simulink model "ideal_defence_zda"  (R2022a)
settings: Solver=VariableStepAuto  StartTime=0.0  StopTime=6  RelTol=1e-3
values from neighbouring files (symbols this model uses):
  A = [zeros(3, 3) eye(3) ... (first row only)    [ideal_defence_zda.m]
  B = [zeros(3, 3); inv(M)]    [ideal_defence_zda.m]
  b = Cp*(A^(r-1))*Bp    [ideal_defence_zda.m]
  H0 = Cp*(A^r)*T0_inv    [ideal_defence_zda.m]
  K = Cp*(A^r)*T1_inv    [ideal_defence_zda.m]
  K0 = [-9 -6]    [ideal_defence_zda.m]
  Ka = (-1)*acker(F0, G0a, [1/tau1 1/tau1 1/tau1 1/tau1])    [ideal_defence_zda.m]
  omega20 = 1.3e-2    (= 0.013)    [ideal_defence_zda.m]
  T0 = [1 0 0 0 0 0 ... (first row only)    [ideal_defence_zda.m]
  T1 = [Cp; Cp*A]    [ideal_defence_zda.m]
settings Model: Creator=edebi  LastModifiedBy=edebi

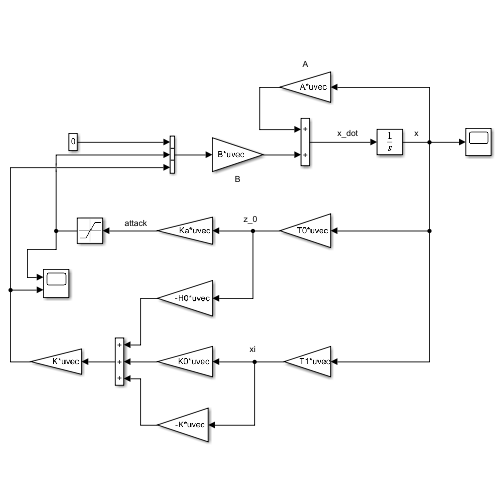
[thumbnail: Simulink's stored preview of the top-level diagram]
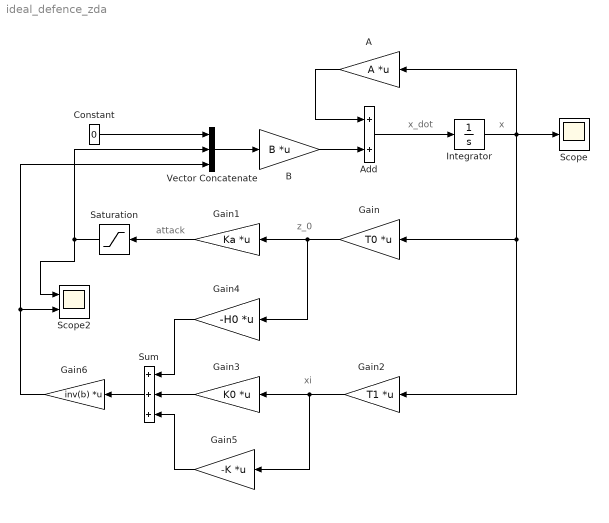
== system ideal_defence_zda ==
  note: xi
  note: attack
  note: z_0
  note: x
  note: x_dot
  A : Gain  Gain=A  Multiplication=Matrix(K*u) (u vector)
  Add : Sum
  B : Gain  Gain=B  Multiplication=Matrix(K*u) (u vector)
  Constant : Constant  Value=0
  Gain : Gain  Gain=T0  Multiplication=Matrix(K*u) (u vector)
  Gain1 : Gain  Gain=Ka  Multiplication=Matrix(K*u) (u vector)
  Gain2 : Gain  Gain=T1  Multiplication=Matrix(K*u) (u vector)
  Gain3 : Gain  Gain=K0  Multiplication=Matrix(K*u) (u vector)
  Gain4 : Gain  Gain=-H0  Multiplication=Matrix(K*u) (u vector)
  Gain5 : Gain  Gain=-K  Multiplication=Matrix(K*u) (u vector)
  Gain6 : Gain  Gain=inv(b)  Multiplication=Matrix(K*u) (u vector)
  Integrator : Integrator  InitialCondition=[0 omega20 0 0 0 0]  ContinuousStateAttributes=['delta1' 'delta2' 'delta3' 'omega1' 'omega2' 'omega3']
  Saturation : Saturate  UpperLimit=0.1  LowerLimit=-0.1
  Scope : Scope
  Scope2 : Scope  NumInputPorts=2
  Sum : Sum  Inputs=+++
  Vector Concatenate : Concatenate  NumInputs=3
  wires:
  Add/1 -> Integrator/1
  Integrator/1 -> Scope/1, A/1, Gain2/1, Gain/1
  A/1 -> Add/1
  B/1 -> Add/2
  Vector Concatenate/1 -> B/1
  Constant/1 -> Vector Concatenate/1
  Gain/1 -> Gain4/1, Gain1/1
  Gain1/1 -> Saturation/1
  Gain2/1 -> Gain5/1, Gain3/1
  Gain3/1 -> Sum/2
  Gain4/1 -> Sum/1
  Gain5/1 -> Sum/3
  Sum/1 -> Gain6/1
  Gain6/1 -> Scope2/2, Vector Concatenate/3
  Saturation/1 -> Scope2/1, Vector Concatenate/2
